simulink model "PMSM_FOC_Controller_Codegen_v2"  (R2024a)
settings: Solver=FixedStepDiscrete  StartTime=0.0  StopTime=0.1  FixedStep=0.0001  RelTol=1e-3
model workspace (MAT data in the model file):
  FOC_AntiWindupGain = Simulink.Parameter
  FOC_AntiWindupGain.Value = 0.20000000298
  FOC_AntiWindupGain.Complexity = 'real'
  FOC_AntiWindupGain.Dimensions = [1 1]
  FOC_AntiWindupGain.DataType = 'single'
  FOC_CurrentPeriod = Simulink.Parameter
  FOC_CurrentPeriod.Value = 9.99999974738e-05
  FOC_CurrentPeriod.Complexity = 'real'
  FOC_CurrentPeriod.Dimensions = [1 1]
  FOC_CurrentPeriod.DataType = 'single'
  FOC_DutyMax = Simulink.Parameter
  FOC_DutyMax.Value = 0.980000019073
  FOC_DutyMax.Complexity = 'real'
  FOC_DutyMax.Dimensions = [1 1]
  FOC_DutyMax.DataType = 'single'
  FOC_DutyMin = Simulink.Parameter
  FOC_DutyMin.Value = 0.019999999553
  FOC_DutyMin.Complexity = 'real'
  FOC_DutyMin.Dimensions = [1 1]
  FOC_DutyMin.DataType = 'single'
  FOC_FluxPM = Simulink.Parameter
  FOC_FluxPM.Value = 0.0500000007451
  FOC_FluxPM.Complexity = 'real'
  FOC_FluxPM.Dimensions = [1 1]
  FOC_FluxPM.DataType = 'single'
  FOC_IqLimit = Simulink.Parameter
  FOC_IqLimit.Value = 8
  FOC_IqLimit.Complexity = 'real'
  FOC_IqLimit.Dimensions = [1 1]
  FOC_IqLimit.DataType = 'single'
  FOC_KiCurrent = Simulink.Parameter
  FOC_KiCurrent.Value = 500
  FOC_KiCurrent.Complexity = 'real'
  FOC_KiCurrent.Dimensions = [1 1]
  FOC_KiCurrent.DataType = 'single'
  FOC_KiSpeed = Simulink.Parameter
  FOC_KiSpeed.Value = 3
  FOC_KiSpeed.Complexity = 'real'
  FOC_KiSpeed.Dimensions = [1 1]
  FOC_KiSpeed.DataType = 'single'
  FOC_KpCurrent = Simulink.Parameter
  FOC_KpCurrent.Value = 1
  FOC_KpCurrent.Complexity = 'real'
  FOC_KpCurrent.Dimensions = [1 1]
  FOC_KpCurrent.DataType = 'single'
  FOC_KpSpeed = Simulink.Parameter
  FOC_KpSpeed.Value = 0.20000000298
  FOC_KpSpeed.Complexity = 'real'
  FOC_KpSpeed.Dimensions = [1 1]
  FOC_KpSpeed.DataType = 'single'
  FOC_Ld = Simulink.Parameter
  FOC_Ld.Value = 0.0010000000475
  FOC_Ld.Complexity = 'real'
  FOC_Ld.Dimensions = [1 1]
  FOC_Ld.DataType = 'single'
  FOC_Lq = Simulink.Parameter
  FOC_Lq.Value = 0.0010000000475
  FOC_Lq.Complexity = 'real'
  FOC_Lq.Dimensions = [1 1]
  FOC_Lq.DataType = 'single'
  FOC_PolePairs = Simulink.Parameter
  FOC_PolePairs.Value = 4
  FOC_PolePairs.Complexity = 'real'
  FOC_PolePairs.Dimensions = [1 1]
  FOC_PolePairs.DataType = 'single'
  FOC_SpeedPeriod = Simulink.Parameter
  FOC_SpeedPeriod.Value = 0.0010000000475
  FOC_SpeedPeriod.Complexity = 'real'
  FOC_SpeedPeriod.Dimensions = [1 1]
  FOC_SpeedPeriod.DataType = 'single'
  FOC_VoltageUtilization = Simulink.Parameter
  FOC_VoltageUtilization.Value = 0.949999988079
  FOC_VoltageUtilization.Complexity = 'real'
  FOC_VoltageUtilization.Dimensions = [1 1]
  FOC_VoltageUtilization.DataType = 'single'
settings Model: Creator=18283  LastModifiedBy=18283
settings OptimizationCC: EnhancedBackFolding=on  PassReuseOutputArgsAs=Individual arguments  ZeroExternalMemoryAtStartup=off  ZeroInternalMemoryAtStartup=off  OptimizeBlockOrder=speed  DifferentSizesBufferReuse=on  OptimizationCustomize=off  EfficientTunableParamExpr=on
settings DebuggingCC: ParameterTunabilityLossMsg=error
settings SFSimCC: MATLABDynamicMemAlloc=off
settings RTWCC: Description=Embedded Coder  SystemTargetFile=ert.tlc  TemplateMakefile=ert_default_tmf
settings CodeAppCC: ForceParamTrailComments=on  IgnoreCustomStorageClasses=off  OperatorAnnotations=on  SimulinkDataObjDesc=on  SFDataObjDesc=on  InsertBlockDesc=on
settings ERTTargetCC: TargetLangStandard=C99 (ISO)  GenerateSampleERTMain=on  SupportNonFinite=off  ERTCustomFileTemplate=example_file_process.tlc

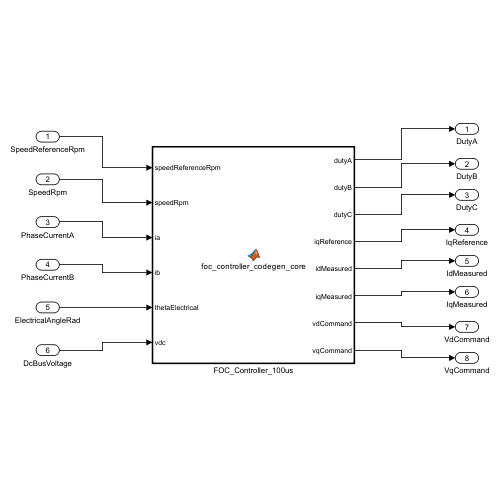
[thumbnail: Simulink's stored preview of the top-level diagram]
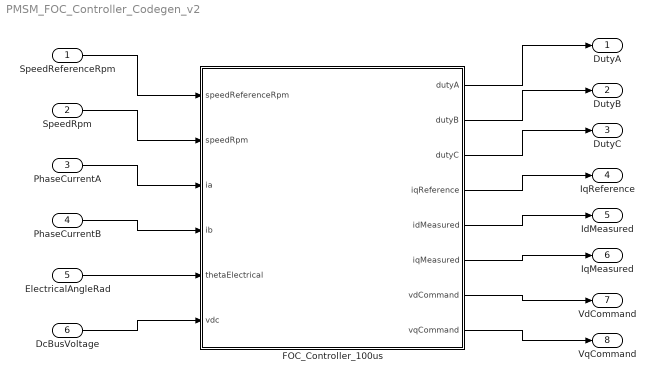
== system PMSM_FOC_Controller_Codegen_v2 ==
  SpeedReferenceRpm : Inport  OutDataTypeStr=single  SampleTime=0.0001
  SpeedRpm : Inport  Port=2  OutDataTypeStr=single  SampleTime=0.0001
  PhaseCurrentA : Inport  Port=3  OutDataTypeStr=single  SampleTime=0.0001
  PhaseCurrentB : Inport  Port=4  OutDataTypeStr=single  SampleTime=0.0001
  ElectricalAngleRad : Inport  Port=5  OutDataTypeStr=single  SampleTime=0.0001
  DcBusVoltage : Inport  Port=6  OutDataTypeStr=single  SampleTime=0.0001
  FOC_Controller_100us : MATLAB Function  TreatAsAtomicUnit=on
  DutyA : Outport  OutDataTypeStr=single
  DutyB : Outport  Port=2  OutDataTypeStr=single
  DutyC : Outport  Port=3  OutDataTypeStr=single
  IqReference : Outport  Port=4  OutDataTypeStr=single
  IdMeasured : Outport  Port=5  OutDataTypeStr=single
  IqMeasured : Outport  Port=6  OutDataTypeStr=single
  VdCommand : Outport  Port=7  OutDataTypeStr=single
  VqCommand : Outport  Port=8  OutDataTypeStr=single
  wires:
  SpeedReferenceRpm/1 -> FOC_Controller_100us/1(speedReferenceRpm)
  SpeedRpm/1 -> FOC_Controller_100us/2(speedRpm)
  PhaseCurrentA/1 -> FOC_Controller_100us/3(ia)
  PhaseCurrentB/1 -> FOC_Controller_100us/4(ib)
  ElectricalAngleRad/1 -> FOC_Controller_100us/5(thetaElectrical)
  DcBusVoltage/1 -> FOC_Controller_100us/6(vdc)
  FOC_Controller_100us/1(dutyA) -> DutyA/1
  FOC_Controller_100us/2(dutyB) -> DutyB/1
  FOC_Controller_100us/3(dutyC) -> DutyC/1
  FOC_Controller_100us/4(iqReference) -> IqReference/1
  FOC_Controller_100us/5(idMeasured) -> IdMeasured/1
  FOC_Controller_100us/6(iqMeasured) -> IqMeasured/1
  FOC_Controller_100us/7(vdCommand) -> VdCommand/1
  FOC_Controller_100us/8(vqCommand) -> VqCommand/1

== matlab function PMSM_FOC_Controller_Codegen_v2/FOC_Controller_100us ==
  data: speedReferenceRpm input; dutyA output; speedRpm input; ia input; ib input; thetaElectrical input; vdc input; dutyB output; dutyC output; iqReference output; idMeasured output; iqMeasured output; vdCommand output; vqCommand output; FOC_CurrentPeriod parameter; FOC_SpeedPeriod parameter; FOC_PolePairs parameter; FOC_Ld parameter; FOC_Lq parameter; FOC_FluxPM parameter; FOC_KpCurrent parameter; FOC_KiCurrent parameter; FOC_KpSpeed parameter; FOC_KiSpeed parameter; FOC_IqLimit parameter; FOC_VoltageUtilization parameter; FOC_AntiWindupGain parameter; FOC_DutyMin parameter; FOC_DutyMax parameter
function [dutyA, dutyB, dutyC, iqReference, idMeasured, iqMeasured, vdCommand, vqCommand] = ...
    foc_controller_codegen_core(speedReferenceRpm, speedRpm, ia, ib, thetaElectrical, vdc, FOC_CurrentPeriod, FOC_SpeedPeriod, FOC_PolePairs, FOC_Ld, FOC_Lq, FOC_FluxPM, FOC_KpCurrent, FOC_KiCurrent, FOC_KpSpeed, FOC_KiSpeed, FOC_IqLimit, FOC_VoltageUtilization, FOC_AntiWindupGain, FOC_DutyMin, FOC_DutyMax)
%#codegen
% Code-generation implementation of the basic PMSM FOC controller.

% These states belong to the deployable controller. The generated
% initialize function resets them when the application starts.
persistent speedIntegrator dIntegrator qIntegrator iqReferenceMemory speedDivider
if isempty(speedIntegrator)
    speedIntegrator = single(0.0);
    dIntegrator = single(0.0);
    qIntegrator = single(0.0);
    iqReferenceMemory = single(0.0);
    speedDivider = uint8(9); % Execute the 1 ms speed loop on the first call.
end

vdc = max(vdc, single(1.0));
sqrtThree = single(1.7320508075688772);
inverseSqrtThree = single(0.5773502691896258);
rpmToRadians = single(0.1047197551196598);

% Clarke and Park transforms.
iAlpha = ia;
iBeta = (ia + single(2.0) * ib) * inverseSqrtThree;
cosTheta = cos(thetaElectrical);
sinTheta = sin(thetaElectrical);
idMeasured = cosTheta * iAlpha + sinTheta * iBeta;
iqMeasured = -sinTheta * iAlpha + cosTheta * iBeta;

% The controller step runs at 100 us; execute the speed PI every ten calls.
if speedDivider >= uint8(9)
    speedDivider = uint8(0);
    speedError = (speedReferenceRpm - speedRpm) * rpmToRadians;
    iqUnsaturated = FOC_KpSpeed * speedError + speedIntegrator;
    iqReference = min(max(iqUnsaturated, -FOC_IqLimit), FOC_IqLimit);
    speedIntegrator = speedIntegrator + ...
        FOC_KiSpeed * FOC_SpeedPeriod * speedError + ...
        FOC_AntiWindupGain * (iqReference - iqUnsaturated);
    speedIntegrator = min(max(speedIntegrator, -FOC_IqLimit), FOC_IqLimit);
else
    speedDivider = speedDivider + uint8(1);
    iqReference = iqReferenceMemory;
end
iqReferenceMemory = iqReference;

% Current PI, dq decoupling and back-EMF feed-forward.
omegaElectrical = speedRpm * rpmToRadians * FOC_PolePairs;
dError = -idMeasured;
qError = iqReference - iqMeasured;
vdRaw = FOC_KpCurrent * dError + dIntegrator - ...
    omegaElectrical * FOC_Lq * iqMeasured;
vqRaw = FOC_KpCurrent * qError + qIntegrator + ...
    omegaElectrical * (FOC_Ld * idMeasured + FOC_FluxPM);

voltageLimit = FOC_VoltageUtilization * vdc * inverseSqrtThree;
magnitudeSquared = vdRaw * vdRaw + vqRaw * vqRaw;
if magnitudeSquared > voltageLimit * voltageLimit
    voltageScale = voltageLimit / sqrt(magnitudeSquared);
else
    voltageScale = single(1.0);
end
vdCommand = vdRaw * voltageScale;
vqCommand = vqRaw * voltageScale;

dIntegrator = dIntegrator + FOC_KiCurrent * FOC_CurrentPeriod * dError + ...
    FOC_AntiWindupGain * (vdCommand - vdRaw);
qIntegrator = qIntegrator + FOC_KiCurrent * FOC_CurrentPeriod * qError + ...
    FOC_AntiWindupGain * (vqCommand - vqRaw);
dIntegrator = min(max(dIntegrator, -voltageLimit), voltageLimit);
qIntegrator = min(max(qIntegrator, -voltageLimit), voltageLimit);

% Inverse Park and centered SVPWM duty ratios.
vAlpha = cosTheta * vdCommand - sinTheta * vqCommand;
vBeta = sinTheta * vdCommand + cosTheta * vqCommand;
va = vAlpha;
vb = single(-0.5) * vAlpha + single(0.5) * sqrtThree * vBeta;
vc = single(-0.5) * vAlpha - single(0.5) * sqrtThree * vBeta;
maximumPhase = max(va, max(vb, vc));
minimumPhase = min(va, min(vb, vc));
commonMode = single(-0.5) * (maximumPhase + minimumPhase);
dutyA = single(0.5) + (va + commonMode) / vdc;
dutyB = single(0.5) + (vb + commonMode) / vdc;
dutyC = single(0.5) + (vc + commonMode) / vdc;
dutyA = min(max(dutyA, FOC_DutyMin), FOC_DutyMax);
dutyB = min(max(dutyB, FOC_DutyMin), FOC_DutyMax);
dutyC = min(max(dutyC, FOC_DutyMin), FOC_DutyMax);
end
